simulink model "CompoundedDCMachine"  (R2013a)
settings: Solver=ode45  StartTime=0.0  StopTime=0.065  RelTol=1e-3
libraries: powerlib x18, simulink x2
settings Model: Creator=Sony  LastModifiedBy=Yooshaa

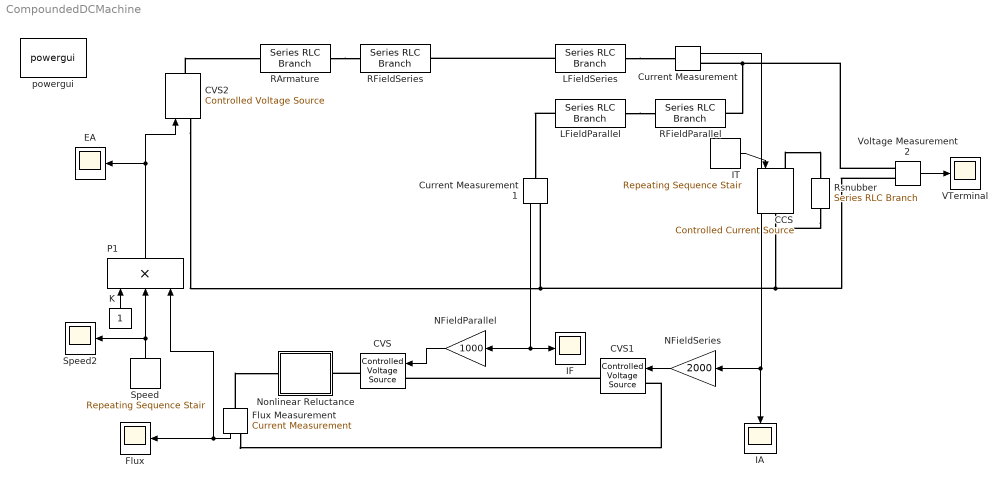
== system CompoundedDCMachine ==
  CCS : powerlib/Electrical Sources/Controlled Current Source  Initialize=off  Source_Type=AC  Amplitude=0  Phase=0  Frequency=0  Measurements=None
  CVS : powerlib/Electrical Sources/Controlled Voltage Source  Initialize=on  Source_Type=DC  Amplitude=50  Phase=0  Frequency=0  Measurements=None
  CVS1 : powerlib/Electrical Sources/Controlled Voltage Source  Initialize=on  Source_Type=DC  Amplitude=50  Phase=0  Frequency=0  Measurements=None
  CVS2 : powerlib/Electrical Sources/Controlled Voltage Source  Initialize=on  Source_Type=DC  Amplitude=50  Phase=0  Frequency=0  Measurements=None
  Current Measurement : powerlib/Measurements/Current Measurement  PhasorSimulation=off  OutputType=Complex  PSBequivalent=0
  Current Measurement1 : powerlib/Measurements/Current Measurement  PhasorSimulation=off  OutputType=Complex  PSBequivalent=0
  EA : Scope
      settings: YMin=0.00937187  YMax=0.0103584  SaveName=EA
  Flux : Scope
      settings: YMin=5.48063e-06  YMax=5.48063e-06  SaveName=ScopeData3
  Flux Measurement : powerlib/Measurements/Current Measurement  PhasorSimulation=off  OutputType=Complex  PSBequivalent=0
  IA : Scope
      settings: YMin=0  YMax=10  SaveName=IA
  IF : Scope
      settings: YMin=0  YMax=20  SaveName=IF
  IT : simulink/Sources/Repeating Sequence Stair  OutValues=[0:0].'  tsamp=0.01  OutMin=[]  OutMax=[]  OutDataTypeStr=double  OutputDataTypeScalingMode=double  OutDataType=fixdt(0,8)  ConRadixGroup=Best Precision: Vector-wise  OutScaling=2^-12
  K : Constant
  LFieldParallel : powerlib/Elements/Series RLC Branch  LConnTagsString=__new0  RConnTagsString=__new0  BranchType=L  Resistance=30  Inductance=1e-3  SetiL0=on  InitialCurrent=1  Capacitance=1e-6  Setx0=off  InitialVoltage=0  Measurements=None
  LFieldSeries : powerlib/Elements/Series RLC Branch  LConnTagsString=__new0  RConnTagsString=__new0  BranchType=L  Resistance=0.02  Inductance=1e-3  SetiL0=on  InitialCurrent=1  Capacitance=1e-6  Setx0=off  InitialVoltage=0  Measurements=None
  NFieldParallel : Gain  Gain=1000
  NFieldSeries : Gain  Gain=2000
  Nonlinear Reluctance : Subsystem  mask{R=1e9, C=1.7e-5}
  P1 : Product  Inputs=3
  RArmature : powerlib/Elements/Series RLC Branch  LConnTagsString=__new0  RConnTagsString=__new0  BranchType=R  Resistance=0.19  Inductance=1e-3  SetiL0=off  InitialCurrent=0  Capacitance=1e-6  Setx0=off  InitialVoltage=0  Measurements=None
  RFieldParallel : powerlib/Elements/Series RLC Branch  LConnTagsString=__new0  RConnTagsString=__new0  BranchType=R  Resistance=20  Inductance=1e-3  SetiL0=off  InitialCurrent=0  Capacitance=1e-6  Setx0=off  InitialVoltage=0  Measurements=None
  RFieldSeries : powerlib/Elements/Series RLC Branch  LConnTagsString=__new0  RConnTagsString=__new0  BranchType=R  Resistance=0.02  Inductance=1e-3  SetiL0=off  InitialCurrent=0  Capacitance=1e-6  Setx0=off  InitialVoltage=0  Measurements=None
  Rsnubber : powerlib/Elements/Series RLC Branch  LConnTagsString=__new0  RConnTagsString=__new0  BranchType=R  Resistance=1e9  Inductance=1e-3  SetiL0=off  InitialCurrent=0  Capacitance=1e-6  Setx0=off  InitialVoltage=0  Measurements=None
  Speed : simulink/Sources/Repeating Sequence Stair  OutValues=[1000:250:2500].'  tsamp=0.01  OutMin=[]  OutMax=[]  OutDataTypeStr=double  OutputDataTypeScalingMode=double  OutDataType=fixdt(0,8)  ConRadixGroup=Best Precision: Vector-wise  OutScaling=2^-12
  Speed2 : Scope
      settings: YMin=1750  YMax=1750  SaveName=RotorSpeed
  VTerminal : Scope
      settings: YMin=0  YMax=150  SaveName=VT
  Voltage Measurement2 : powerlib/Measurements/Voltage Measurement  PhasorSimulation=off  OutputType=Complex  PSBequivalent=0
  powergui : powerlib/powergui  Priority=1  SimulationMode=Discrete  SolverType=Backward Euler  SampleTime=1e-7  frequency=60  SPID=off  DisableSnubberDevices=off  DisableRonSwitches=off  DisableVfSwitches=off  SwTol=0  Interpol=off  DisplayEquations=off  frequencyindice=0  Pbase=100e6  ErrMax=1e-4  Iterations=50  UnitsV=kV  UnitsW=MW  FunctionMessages=off  echomessages=off  HookPort=off  EnableUseOfTLC=off  x0status=steady  RestoreLinks=warning  ResistiveCurrentMeasurement=off  Frange=[0:2:500]  Ylog=off  Xlog=on  ShowGrid=off  save=off  variable=ZData  ZoomFFT=off  StartTime=0.0  cycles=1  DisplayStyle=1  fundamental=60  FreqAxis=off  MaxFrequency=1000  frequencyindicesteady=1  RmsSteady=1  display=off  Ts=0  methode=off
  wires:
  Current Measurement/1 -> IA/1, NFieldSeries/1
  Current Measurement1/1 -> IF/1, NFieldParallel/1
  NFieldParallel/1 -> CVS/1
  NFieldSeries/1 -> CVS1/1
  Flux Measurement/1 -> Flux/1, P1/3
  K/1 -> P1/1
  Speed/1 -> Speed2/1, P1/2
  P1/1 -> CVS2/1, EA/1
  Voltage Measurement2/1 -> VTerminal/1
  IT/1 -> CCS/1
  connections:
  Voltage Measurement2/LConn1 -- Current Measurement/RConn1 -- RFieldParallel/LConn1
  Voltage Measurement2/LConn2 -- Rsnubber/RConn1 -- CCS/RConn1 -- CVS2/LConn1 -- Current Measurement1/RConn1
  LFieldParallel/RConn1 -- Current Measurement1/LConn1
  RArmature/RConn1 -- RFieldSeries/LConn1
  LFieldSeries/RConn1 -- Current Measurement/LConn1
  CVS2/RConn1 -- RArmature/LConn1
  Flux Measurement/RConn1 -- CVS1/LConn1
  CVS1/RConn1 -- CVS/LConn1
  CVS/RConn1 -- Nonlinear Reluctance/LConn1
  LFieldSeries/LConn1 -- RFieldSeries/RConn1
  LFieldParallel/LConn1 -- RFieldParallel/RConn1
  Flux Measurement/LConn1 -- Nonlinear Reluctance/RConn1
  CCS/LConn1 -- Rsnubber/LConn1

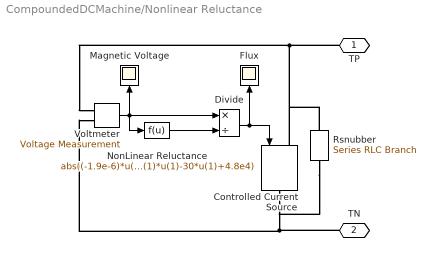
== system CompoundedDCMachine/Nonlinear Reluctance ==
  Controlled Current Source : powerlib/Electrical Sources/Controlled Current Source  Initialize=on  Source_Type=AC  Amplitude=0  Phase=0  Frequency=0  Measurements=None
  Divide : Product  Inputs=*/
  Flux : Scope
      settings: YMin=2.75e-06  YMax=8.5e-06  SaveName=PermeanceFlux
  Magnetic Voltage : Scope
      settings: YMin=0  YMax=10000  SaveName=PermeanceVm
  NonLinear Reluctance : Fcn  Expr=abs((-1.9e-6)*u(1)*u(1)*u(1)+0.024*u(1)*u(1)-30*u(1)+4.8e4)
  Rsnubber : powerlib/Elements/Series RLC Branch  LConnTagsString=__new0  RConnTagsString=__new0  BranchType=R  Resistance=R  Inductance=1e-3  SetiL0=off  InitialCurrent=0  Capacitance=1e-6  Setx0=off  InitialVoltage=0  Measurements=None
  Voltmeter : powerlib/Measurements/Voltage Measurement  PhasorSimulation=off  OutputType=Complex  PSBequivalent=0
  TP : PMIOPort  Port=1  Side=Left
  TN : PMIOPort  Port=2  Side=Right
  wires:
  Voltmeter/1 -> Divide/1, Magnetic Voltage/1, NonLinear Reluctance/1
  Divide/1 -> Flux/1, Controlled Current Source/1
  NonLinear Reluctance/1 -> Divide/2
  connections:
  TN/RConn1 -- Voltmeter/LConn2 -- Rsnubber/RConn1 -- Controlled Current Source/RConn1
  TP/RConn1 -- Rsnubber/LConn1 -- Controlled Current Source/LConn1 -- Voltmeter/LConn1
